simulink model "SAD_projectSamu"  (R2023b)
settings: Solver=ode4  StartTime=t0  StopTime=1000  FixedStep=t_step  RelTol=1e-3
model workspace (MAT data in the model file):
  N_order = 1
values from neighbouring files (symbols this model uses):
  A1 = importdata("igrfSg.txt")    [SAD_project_code.m]
  A2 = importdata("igrfSh.txt")    [SAD_project_code.m]
  A_1 = area_face(1)    [SAD_project_code.m]
  A_2 = area_face(2)    [SAD_project_code.m]
  A_3 = area_face(3)    [SAD_project_code.m]
  A_4 = area_face(4)    [SAD_project_code.m]
  A_5 = area_face(5)    [SAD_project_code.m]
  A_6 = area_face(6)    [SAD_project_code.m]
  alpha = [1/6 5/6]    [SAD_project_code.m]
  ARW = ARW*[1 1 1]'    [SAD_project_code.m]
  bias = bias*[1 1 1]'    [SAD_project_code.m]
  DCM_eci_per = rotationMatrix(rad2deg(i),rad2deg(OM), rad2deg(om))    [SAD_project_code.m]
  e = 0.0011241    [SAD_project_code.m]
  FS = 50000e-9    (= 5e-05)    [SAD_project_code.m]
  H0 = [g_10 g_11 h_11]'    [SAD_project_code.m]
  h_r_0 = [0,0,0]'    [SAD_project_code.m]
  horizon_cone_limit = deg2rad(350)    [SAD_project_code.m]
  I = 5/12.*diag([Ix Iy Iz])    [SAD_project_code.m]
  i = deg2rad(97.55)    [SAD_project_code.m]
  I_inv = inv(I)    [SAD_project_code.m]
  I_RW = 1e-2    (= 0.01)    [SAD_project_code.m]
  I_vector_RW = [I_RW I_RW I_RW]'    [SAD_project_code.m]
  inc_tot = sqrt(inc_lin^2 + inc_acc^2)    [SAD_project_code.m]
  InitialTrueAnomalyOfEarth = 0    [SAD_project_code.m]
  j_b = [0.001 0.005 0.001]'    [SAD_project_code.m]
  K1_point = lqr(A, B, Q, R)    [SAD_project_code.m]
  K1_slew = lqr(A,B, Q, R)    [SAD_project_code.m]
  K2_point = K1_point.^2/2    [SAD_project_code.m]
  K2_slew = K1_slew.^2/2    [SAD_project_code.m]
  K_detumbling = lqr(A,B,Q,R)    [SAD_project_code.m]
  matrix_RW_config = eye(3)    [SAD_project_code.m]
  matrix_RW_config_inv = inv(matrix_RW_config)    [SAD_project_code.m]
  mu_E = astroConstants(13)    [SAD_project_code.m]
  N_1 = BODY(1,:)    [SAD_project_code.m]
  N_2 = BODY(2,:)    [SAD_project_code.m]
  N_3 = BODY(3,:)    [SAD_project_code.m]
  N_4 = BODY(4,:)    [SAD_project_code.m]
  N_5 = BODY(5,:)    [SAD_project_code.m]
  N_6 = BODY(6,:)    [SAD_project_code.m]
  n_e = sqrt(mu_E/a^3)    [SAD_project_code.m]
  om = deg2rad(206.3209)    [SAD_project_code.m]
  OM = deg2rad(50.7464)    [SAD_project_code.m]
  p = a*(1-e^2)    [SAD_project_code.m]
  q0 = [0.1, -0.7, 0.51, 0.41]    [SAD_project_code.m]
  r_1 = r(1,:)    [SAD_project_code.m]
  r_2 = r(2,:)    [SAD_project_code.m]
  r_3 = r(3,:)    [SAD_project_code.m]
  r_4 = r(4,:)    [SAD_project_code.m]
  r_5 = r(5,:)    [SAD_project_code.m]
  r_6 = r(6,:)    [SAD_project_code.m]
  R_E = astroConstants(23)    [SAD_project_code.m]
  rho_d1 = 0.1    [SAD_project_code.m]
  rho_d2 = 0.1    [SAD_project_code.m]
  rho_d3 = 0.1    [SAD_project_code.m]
  rho_d4 = 0.1    [SAD_project_code.m]
  rho_d5 = 0.1    [SAD_project_code.m]
  rho_d6 = 0.1    [SAD_project_code.m]
  rho_s1 = rho_s(1)    [SAD_project_code.m]
  rho_s2 = rho_s(2)    [SAD_project_code.m]
  rho_s3 = rho_s(3)    [SAD_project_code.m]
  rho_s4 = rho_s(4)    [SAD_project_code.m]
  rho_s5 = rho_s(5)    [SAD_project_code.m]
  rho_s6 = rho_s(6)    [SAD_project_code.m]
  t_step = 0.01    [SAD_project_code.m]
  th0 = deg2rad(0)    [SAD_project_code.m]
  timeoflaunch = date2mjd2000(date0)    [SAD_project_code.m]
  torque_max = 0.8    [SAD_project_code.m]
  ts_sensor = 5*t_step    (= 0.05)    [SAD_project_code.m]
  w0 = [wx0 wy0 wz0]'    [SAD_project_code.m]
  w0_RW = [0 0 0]    [SAD_project_code.m]
  w_E = deg2rad(15.04)/60/60    [SAD_project_code.m]
  wMax_RW = 2*pi * RPM_max_RW / 60    (= 527.263967027)    [SAD_project_code.m]
libraries: matrix_library x43, dspindex x6, simulink x5, simulink_extras x4, sharedtransform x4, aerolibutil x2, vrlib x2, dspinverses x1
(part 1 of 4)
settings Model: PacingRate=0.100000  Creator=samue  LastModifiedBy=samue

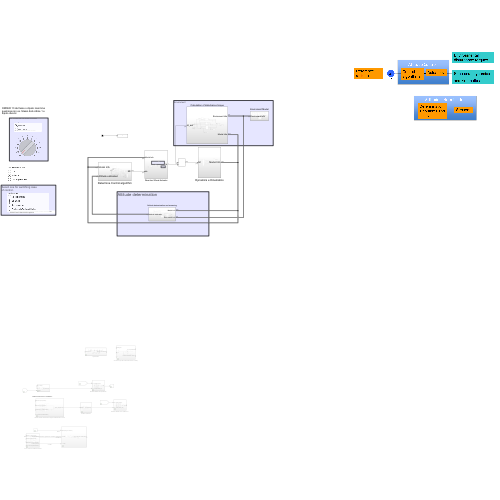
[thumbnail: Simulink's stored preview of the top-level diagram]
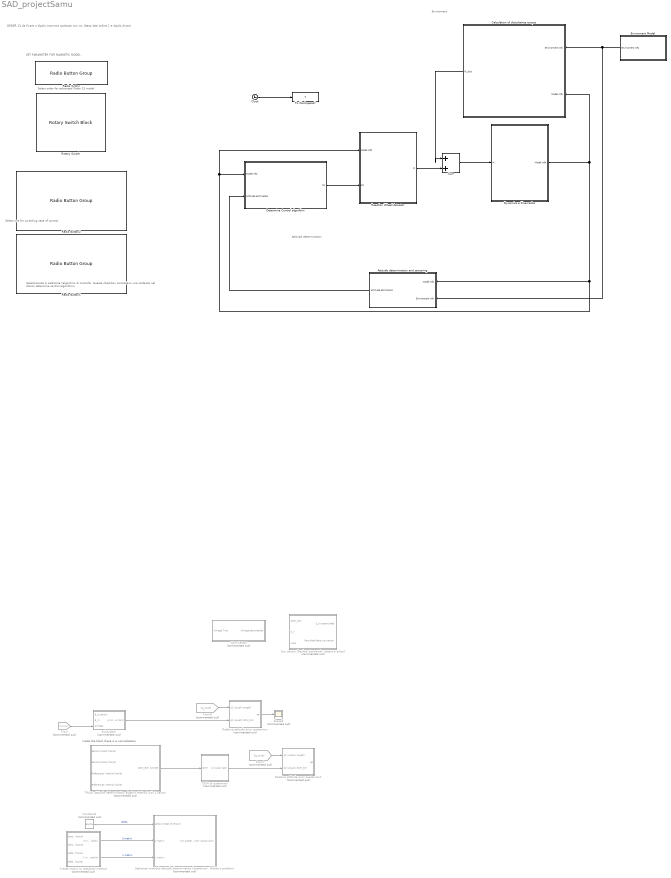
== system SAD_projectSamu ==
  note: ORDER 13 da fixare o dipolo insomma qualcosa non va. Stessi dati ordine 1 e dipolo diversi
  note: Select order for advanced Order 13 model
  note: SET PARAMETER FOR MAGNETIC MODEL
  note: Selezionando si seleziona l'algoritmo di controllo. Queste checkbox controllano una costante nel blocco determine control algorithmù
  note: Select one for switching case
      | of control.
  note: Attitude determination
  note: inside the block there is a normalisation
  note: Enviroment
  Attitude determination and sensoring : Subsystem
  Calculation of disturbance torque : Subsystem
  Clock : Clock
  Constant1 : Constant  Commented=on  Value=alpha
  Create matrix to statistical method : Subsystem  Commented=on
  DCM to quaternion : Subsystem  Commented=on
  Determine Control algorithm : Subsystem
  Dynamics e Kinematics : Subsystem
  Enviroment Model : Subsystem
  From : From  Commented=on  GotoTag=w_true
  From7 : From  Commented=on  GotoTag=q_true
  From8 : From  Commented=on  GotoTag=q_true
  Gyro Sensor : Subsystem  Commented=on
  Radio Button : RadioButtonGroup  LabelPosition=Hide  SelectedLabel=Dipole model  ButtonGroupName=Magnetic field
      settings: Values={{'Dipole model', 'Order 13 model'}, [0 1]}
  Radio Button1 : RadioButtonGroup  LabelPosition=Hide  SelectedLabel=De-tumble  ButtonGroupName=Control Mode
      settings: Values={{'No control mode', 'De-tumble', 'Slew maneuver', 'Pointing with 3 axis stabilization'}, [0 1 2 3]}
  Radio Button2 : RadioButtonGroup  LabelPosition=Hide  SelectedLabel=Statisitcal  ButtonGroupName=Attitude Determination
      settings: Values={{'Triad', 'Statisitcal', 'Only Magnetometer'}, [0 2 1]}
  Reaction Wheel Actuator : Subsystem
  Relative attitude error quaternion : Subsystem  Commented=on
  Relative attitude error quaternion1 : Subsystem  Commented=on
  Rotary Switch : RotarySwitchBlock  LabelPosition=Hide
      settings: Values={{'1', '2', '3', '4', '5', '6', '7', '8', '9', '10', '11', '12', '13'}, [1 2 3 4 5 6 7 8 9 10 11 12 13]}
  Scope3 : Scope  Commented=on
  "Statistical methods attitude determination (quaternion  Wabha’s problem) " : Subsystem  Commented=on
  Subsystem : Subsystem  Commented=on
  Sum : Sum  Inputs=|++
  Sun sensor (Da fare sistmando vettore e eclissi) : Subsystem  Commented=on
  TRIAD: Attitude determination algebric Method with 2 sensor : Subsystem  Commented=on
  To Workspace7 : ToWorkspace  VariableName=t  SampleTime=-1
  wires:
  Clock/1 -> To Workspace7/1
  Create matrix to statistical method/2(V matrix (inertia)) -> "Statistical methods attitude determination (quaternion  Wabha’s problem) "/3(v matrix)  "V matrix"
  Constant1/1 -> "Statistical methods attitude determination (quaternion  Wabha’s problem) "/1(alpha (weigh of sensor))  "alpha"
  Create matrix to statistical method/1(S matrix (body)) -> "Statistical methods attitude determination (quaternion  Wabha’s problem) "/2(s matrix)  "S matrix"
  TRIAD: Attitude determination algebric Method with 2 sensor/1(DCM_B/N  Att Det) -> DCM to quaternion/1(DCM)
  From/1 -> Subsystem/3(Omega)
  From8/1 -> Relative attitude error quaternion/1(q1 (usually target))
  Subsystem/1(q (scalar last)) -> Relative attitude error quaternion/2(q2 (usually DCM_bn))
  Relative attitude error quaternion/1(qe) -> Scope3/1
  DCM to quaternion/1(q (scalar last)) -> Relative attitude error quaternion1/2(q2 (usually DCM_bn))
  From7/1 -> Relative attitude error quaternion1/1(q1 (usually target))
  Reaction Wheel Actuator/1(M) -> Sum/2
  Sum/1 -> Dynamics e Kinematics/1(M)
  Enviroment Model/1(Enviroment Info) -> Attitude determination and sensoring/2(Enviroment info), Calculation of disturbance torque/1(Enviroment Info)
  Calculation of disturbance torque/1(M_dist) -> Sum/1
  Determine Control algorithm/1(Mc) -> Reaction Wheel Actuator/2(Mc)
  Dynamics e Kinematics/1(Model Info) -> Calculation of disturbance torque/2(Model Info), Determine Control algorithm/1(Model Info), Reaction Wheel Actuator/1(Model Info), Attitude determination and sensoring/1(Model Info)
  Attitude determination and sensoring/1(Attitude estimation) -> Determine Control algorithm/2(Attitude estimated)

== system SAD_projectSamu/Attitude determination and sensoring ==
  Model Info : Inport
  Enviroment info : Inport  Port=2
  Bus Selector : BusSelector  OutputSignals=B_N,r_n
  Bus Selector1 : BusSelector  OutputSignals=w_b true,DCM_BN,q_b True
  Demux : Demux
  Demux1 : Demux  Outputs=3
  Display : Display
  Horizon Sensor : Subsystem
  MAG-3  Magnetometer1 : Subsystem
  Relative attitude error quaternion2 : Subsystem
  Reshape3 : Reshape
  "SCOPE ERROR ATTITUTE ESTIMATION RESPECT TO DCM_BN TRUE " : Scope  NumInputPorts=4
  "SCOPE ERROR w estimated RESPECT TO w TRUE " : Scope  NumInputPorts=3
  Subsystem1 : Subsystem
  Subtract : Sum  Inputs=+-
  To Workspace5 : ToWorkspace  VariableName=b_sensor  SampleTime=-1
  Transpose : Math  Operator=transpose
  Out Bus Element2 : Outport  PortName=Attitude estimation  Element=q estimated
  Out Bus Element1 : Outport  PortName=Attitude estimation  Element=w estimated
  wires:
  MAG-3  Magnetometer1/2(B_n) -> Subsystem1/3(B_N)
  Horizon Sensor/3(Falg IsEarthVisible) -> Subsystem1/6(Flag IsEarthVisible)
  Horizon Sensor/1(Perturbed data Horizon) -> Subsystem1/4(Horizon_b sensor)  "R_b perturbed sensor"
  Horizon Sensor/2(R_N Horizon) -> Subsystem1/5(Horizon_N)
  MAG-3  Magnetometer1/1(B_b perturbed sensor) -> Subsystem1/2(B_b sensor), Reshape3/1
  Bus Selector/1 -> Transpose/1  "<B_N>"
  Enviroment info/1 -> Bus Selector/1
  Bus Selector/2 -> Horizon Sensor/2(R_N)  "<r_n>"
  Bus Selector1/2 -> Horizon Sensor/1(DCM_B/N), MAG-3  Magnetometer1/1(DCM_B/N)  "<DCM_BN>"
  Reshape3/1 -> To Workspace5/1
  Model Info/1 -> Bus Selector1/1
  Transpose/1 -> MAG-3  Magnetometer1/2(B_N)
  Demux/1 -> "SCOPE ERROR ATTITUTE ESTIMATION RESPECT TO DCM_BN TRUE "/1
  Demux/3 -> "SCOPE ERROR ATTITUTE ESTIMATION RESPECT TO DCM_BN TRUE "/3
  Relative attitude error quaternion2/1(qe) -> Demux/1
  Demux/4 -> "SCOPE ERROR ATTITUTE ESTIMATION RESPECT TO DCM_BN TRUE "/4
  Bus Selector1/1 -> Subtract/1, Subsystem1/1(w_true)  "<w_b true>"
  Demux/2 -> "SCOPE ERROR ATTITUTE ESTIMATION RESPECT TO DCM_BN TRUE "/2
  Bus Selector1/3 -> Relative attitude error quaternion2/1(q1 (usually Target))  "<q_b True>"
  Subtract/1 -> Demux1/1
  Demux1/2 -> "SCOPE ERROR w estimated RESPECT TO w TRUE "/2
  Demux1/1 -> "SCOPE ERROR w estimated RESPECT TO w TRUE "/1
  Demux1/3 -> "SCOPE ERROR w estimated RESPECT TO w TRUE "/3
  Subsystem1/1(q estimated) -> Out Bus Element2/1, Display/1, Relative attitude error quaternion2/2(q2 (Estimated))
  Subsystem1/2(w estimated) -> Out Bus Element1/1, Subtract/2

== system SAD_projectSamu/Calculation of disturbance torque ==
  Enviroment Info : Inport
  Model Info : Inport  Port=2
  Bus Selector : BusSelector  OutputSignals=r_n,S_N,B_N
  Bus Selector1 : BusSelector  OutputSignals=DCM_BL,DCM_BN
  Constant : Constant  Value=I
  Extract Diagonal : matrix_library/Extract Diagonal
      settings: LibrarySourceBlock=|
      | simulink/Matrix
      | Operations/Extract Diagonal
  M of gravity gradient1 : Subsystem
  Magnetic Torque : Subsystem
  Matrix Multiply : Product  Multiplication=Matrix(*)
  Reshape{,1..2,4} (4 alike) : Reshape
  Solar pressure on 6 faces : Subsystem
  Sum : Sum  Inputs=|+++
  Terminator : Terminator
  To Workspace1 : ToWorkspace  VariableName=M_b  SampleTime=-1
  To Workspace2 : ToWorkspace  VariableName=M_dist  SampleTime=-1
  To Workspace3 : ToWorkspace  VariableName=M_GG  SampleTime=-1
  To Workspace6 : ToWorkspace  VariableName=bn  SampleTime=-1
  To Workspace8 : ToWorkspace  VariableName=M_SRP  SampleTime=-1
  j_b : Constant  Value=j_b
  M_dist : Outport
  wires:
  j_b/1 -> Magnetic Torque/1(j_b)
  Magnetic Torque/1(M_b) -> Sum/3, Reshape1/1
  Sum/1 -> Reshape2/1, M_dist/1
  Reshape/1 -> To Workspace8/1
  Reshape1/1 -> To Workspace1/1
  M of gravity gradient1/1(GravityGradient_M) -> To Workspace3/1, Sum/1
  Solar pressure on 6 faces/2(Ftot_SP) -> Terminator/1
  Solar pressure on 6 faces/1(Mtot_SP) -> Reshape/1
  Extract Diagonal/1 -> M of gravity gradient1/1(Inertia Vector)
  Reshape4/1 -> To Workspace6/1
  Matrix Multiply/1 -> Reshape4/1, Magnetic Torque/2(B_b)  "B_b"
  Enviroment Info/1 -> Bus Selector/1
  Constant/1 -> Extract Diagonal/1
  Bus Selector/1 -> M of gravity gradient1/3(r_N), Solar pressure on 6 faces/2("r_N ")  "<r_n>"
  Bus Selector/2 -> Solar pressure on 6 faces/3(S_N)  "<S_N>"
  Bus Selector/3 -> Matrix Multiply/1  "<B_N>"
  Model Info/1 -> Bus Selector1/1
  Bus Selector1/2 -> Matrix Multiply/2, Solar pressure on 6 faces/1(DCM_BN)  "<DCM_BN>"
  Bus Selector1/1 -> M of gravity gradient1/2(A_B/L)  "<DCM_BL>"
  Reshape2/1 -> To Workspace2/1

== system SAD_projectSamu/Create matrix to statistical method ==
  Sensor1 (body frame) : Inport
  Sensor2 (body frame) : Inport  Port=2
  Reference1 (Inertial frame) : Inport  Port=3
  Reference2 (Inertial frame) : Inport  Port=4
  Matrix Concatenate1 : Concatenate  Mode=Multidimensional array  ConcatenateDimension=2
  Matrix Concatenate2 : Concatenate  Mode=Multidimensional array  ConcatenateDimension=2
  Normalize Vector1 : Subsystem
  Normalize Vector2 : Subsystem
  Normalize Vector3 : Subsystem
  Normalize Vector4 : Subsystem
  S matrix (body) : Outport
  V matrix (inertia) : Outport  Port=2
  wires:
  Matrix Concatenate1/1 -> V matrix (inertia)/1
  Normalize Vector1/1(Versor) -> Matrix Concatenate2/1
  Normalize Vector2/1(Versor) -> Matrix Concatenate2/2
  Normalize Vector4/1(Versor) -> Matrix Concatenate1/2
  Normalize Vector3/1(Versor) -> Matrix Concatenate1/1
  Matrix Concatenate2/1 -> S matrix (body)/1
  Reference1 (Inertial frame)/1 -> Normalize Vector3/1(Vector)
  Reference2 (Inertial frame)/1 -> Normalize Vector4/1(Vector)
  Sensor1 (body frame)/1 -> Normalize Vector1/1(Vector)
  Sensor2 (body frame)/1 -> Normalize Vector2/1(Vector)

== system SAD_projectSamu/DCM to quaternion ==
  DCM : Inport
  Constant : Constant
  Divide : Product  Inputs=*/
  Extract Diagonal : matrix_library/Extract Diagonal
      settings: LibrarySourceBlock=|
      | simulink/Matrix
      | Operations/Extract Diagonal
  Gain : Gain  Gain=0.5
  Gain1 : Gain  Gain=[0 0 0; 0 0 1; 0 -1 0]
  Gain2 : Gain  Gain=[0 0 -1; 0 0 0; 1 0 0]
  Gain3 : Gain  Gain=[0 1 0; -1 0 0; 0 0 0]
  Gain4 : Gain  Gain=4
  Normalize Vector1 : Subsystem
  Sqrt : Sqrt
  Sum : Sum  Inputs=|++
  Sum of Elements{,1..3} (4 alike) : Sum  Inputs=+
  Vector Concatenate : Concatenate  NumInputs=3
  Vector Concatenate1 : Concatenate
  q (scalar last) : Outport
  wires:
  Extract Diagonal/1 -> Sum of Elements/1
  Sum of Elements/1 -> Sum/1
  Constant/1 -> Sum/2
  Sum/1 -> Sqrt/1
  Sqrt/1 -> Gain/1
  DCM/1 -> Gain1/1, Gain2/1, Gain3/1, Extract Diagonal/1
  Gain2/1 -> Sum of Elements1/1
  Sum of Elements1/1 -> Vector Concatenate/2
  Gain1/1 -> Sum of Elements2/1
  Sum of Elements2/1 -> Vector Concatenate/1
  Sum of Elements3/1 -> Vector Concatenate/3
  Gain3/1 -> Sum of Elements3/1
  Vector Concatenate/1 -> Divide/1
  Gain/1 -> Vector Concatenate1/2, Gain4/1
  Gain4/1 -> Divide/2
  Divide/1 -> Vector Concatenate1/1
  Vector Concatenate1/1 -> Normalize Vector1/1(Vector)
  Normalize Vector1/1(Versor) -> q (scalar last)/1

== system SAD_projectSamu/Determine Control algorithm ==
  Model Info : Inport
  Attitude estimated : Inport  Port=2
  Bus Selector : BusSelector  OutputSignals=q estimated
  Constant2 : Constant
  Demux : Demux
  Demux4 : Demux
  Demux5 : Demux
  Merge : Merge  Inputs=4
  Merge1 : Merge
  Mux{4..7} (4 alike) : Mux  Inputs=2
  Relative attitude error quaternion3 : Subsystem
  Saturation : Saturate  LowerLimit=-torque_max
  Scope : Scope  NumInputPorts=4
  Scope1 : Scope  NumInputPorts=4
  Switch Case : SwitchCase  CaseConditions={1,2,3}
  Switch Case Action 3 axis stabilization Algorithm : Subsystem  TreatAsAtomicUnit=on
  Switch Case Action Detumle Algorithm : Subsystem  TreatAsAtomicUnit=on
  Switch Case Action Mc = 0 : Subsystem  TreatAsAtomicUnit=on
  Switch Case Action Slew Maneuver Algorithm : Subsystem  TreatAsAtomicUnit=on
  Zero-Order Hold : ZeroOrderHold  SampleTime=5*ts_sensor
  Zero-Order Hold1 : ZeroOrderHold  SampleTime=5*ts_sensor
  Mc : Outport
  wires:
  Switch Case/2 -> Switch Case Action Slew Maneuver Algorithm/Action  "slew maneuver"
  Switch Case/1 -> Switch Case Action Detumle Algorithm/Action  "Detumble case"
  Switch Case Action Slew Maneuver Algorithm/1(Mc) -> Merge/2
  Switch Case/3 -> Switch Case Action 3 axis stabilization Algorithm/Action  "pointing with 3 axis stabilization"
  Switch Case Action Mc = 0/1(Output) -> Merge/4
  Constant2/1 -> Switch Case/1
  Switch Case Action Detumle Algorithm/1(Out1) -> Merge/1
  Switch Case Action 3 axis stabilization Algorithm/1(Mc) -> Merge/3
  Switch Case/4 -> Switch Case Action Mc = 0/Action  "Default: Contol moment == 0"
  Merge/1 -> Saturation/1  "Control Moment"
  Model Info/1 -> Zero-Order Hold1/1
  Attitude estimated/1 -> Zero-Order Hold/1
  Demux4/1 -> Mux4/2
  Demux4/4 -> Mux7/2
  Demux5/3 -> Mux6/1
  Demux5/4 -> Mux7/1
  Mux5/1 -> Scope1/2
  Merge1/1 -> Demux5/1, Relative attitude error quaternion3/1(q1 (usually Target))  "q target"
  Mux6/1 -> Scope1/3
  Mux7/1 -> Scope1/4
  Demux4/3 -> Mux6/2
  Demux5/2 -> Mux5/1
  Demux4/2 -> Mux5/2
  Mux4/1 -> Scope1/1
  Demux5/1 -> Mux4/1
  Switch Case Action 3 axis stabilization Algorithm/2(q target) -> Merge1/1
  Bus Selector/1 -> Relative attitude error quaternion3/2(q2 (Estimated)), Demux4/1  "<q estimated>"
  Switch Case Action Slew Maneuver Algorithm/2(q target) -> Merge1/2
  Relative attitude error quaternion3/1(qe) -> Demux/1
  Demux/1 -> Scope/1
  Demux/2 -> Scope/2
  Demux/3 -> Scope/3
  Demux/4 -> Scope/4
  Zero-Order Hold1/1 -> Switch Case Action Slew Maneuver Algorithm/1(Model info), Switch Case Action 3 axis stabilization Algorithm/1(Model info)
  Zero-Order Hold/1 -> Switch Case Action 3 axis stabilization Algorithm/2(InBus), Switch Case Action Detumle Algorithm/1(Attitude estimated), Switch Case Action Slew Maneuver Algorithm/2(Attitude estimated), Bus Selector/1
  Saturation/1 -> Mc/1

== system SAD_projectSamu/Dynamics e Kinematics ==
  M : Inport
  Attitude error GG : Subsystem
  Constant : Constant  Value=I_inv
  Constant6 : Constant  Value=q0
  DCM composition from quaternions 1 : Subsystem  AncestorBlock=LibrarySAD5/DCM composition from quaternions
  Inertia Matrix : Constant  Value=I  VectorParams1D=off
  Initial Condition W : Constant  Value=w0
  Kinematics quaternion2 : Subsystem
  Reshape : Reshape
  Reshape1 : Reshape
  Single spin dynamics : Subsystem  AncestorBlock=My_library/Single spin dynamics
  Terminator1 : Terminator
  To Workspace2 : ToWorkspace  VariableName=wb  SampleTime=-1
  To Workspace4 : ToWorkspace  VariableName=w  SampleTime=-1
  Transpose : Math  Operator=transpose
  Out Bus Element : Outport  PortName=Model Info  Element=w_b true
  Out Bus Element1 : Outport  PortName=Model Info  Element=Ang vel error
  Out Bus Element2 : Outport  PortName=Model Info  Element=DCM_BL
  Out Bus Element3 : Outport  PortName=Model Info  Element=q_b True
  Out Bus Element4 : Outport  PortName=Model Info  Element=DCM_BN
  Out Bus Element5 : Outport  PortName=Model Info  Element=A_L/N
  wires:
  Single spin dynamics/1(Omega) -> Transpose/1, Attitude error GG/1(w), Reshape1/1, Kinematics quaternion2/1(omega)  "w_b true"
  M/1 -> Single spin dynamics/4(M)
  Constant/1 -> Single spin dynamics/1(Inertia matrix inverse)
  Inertia Matrix/1 -> Single spin dynamics/2(Inertia matrix)
  Initial Condition W/1 -> Single spin dynamics/3(Omega_0)
  Constant6/1 -> Kinematics quaternion2/2(q0)
  Kinematics quaternion2/1(q) -> DCM composition from quaternions 1/1(q(4x1)), Out Bus Element3/1  "q_b True"
  Reshape1/1 -> To Workspace4/1
  Kinematics quaternion2/2(q^(-1)) -> Terminator1/1
  DCM composition from quaternions 1/1(DCM) -> Out Bus Element4/1, Attitude error GG/2(DCM_B/N)  "DCM_BN"
  Attitude error GG/1(Ang Vel Error) -> Out Bus Element1/1, Reshape/1  "Ang vel error"
  Attitude error GG/2(DCM_B/L) -> Out Bus Element2/1
  Reshape/1 -> To Workspace2/1
  Transpose/1 -> Out Bus Element/1
  Attitude error GG/3(A_L/N) -> Out Bus Element5/1

== system SAD_projectSamu/Enviroment Model ==
  Bus Creator : BusCreator  Inputs=3
  Constant4 : Constant  Value=th0
  Magnetic Field : Subsystem
  Sun Position in Earth Centred Equatorial Inertial RF : Subsystem
  To Workspace : ToWorkspace  VariableName=r_n  SampleTime=-1
  two-body Keplerian dynamics ECI : Subsystem
  Enviroment Info : Outport
  wires:
  Constant4/1 -> two-body Keplerian dynamics ECI/1(th0)
  Sun Position in Earth Centred Equatorial Inertial RF/1(s_N) -> Bus Creator/2  "S_N"
  two-body Keplerian dynamics ECI/1(r_n) -> Magnetic Field/1(r_N), Bus Creator/1, To Workspace/1  "r_n"
  Magnetic Field/1(B_N) -> Bus Creator/3  "B_N"
  Bus Creator/1 -> Enviroment Info/1

== system SAD_projectSamu/Gyro Sensor ==
  Omega True : Inport
  Band-Limited White Noise : simulink/Sources/Band-Limited White Noise  Cov=[0.00001]  Ts=0.1  seed=[23341]
  Constant : Constant  Value=ARW  VectorParams1D=off
  Constant1 : Constant  Value=bias  VectorParams1D=off
  Sum : Sum  Inputs=|++
  Sum1 : Sum  Inputs=|++
  Sum2 : Sum  Inputs=|++
  Zero-Order Hold : ZeroOrderHold  SampleTime=-1
  Omega perturbated : Outport
  wires:
  Zero-Order Hold/1 -> Sum/1
  Sum2/1 -> Omega perturbated/1
  Sum1/1 -> Sum2/1
  Sum/1 -> Sum1/1
  Omega True/1 -> Zero-Order Hold/1
  Constant1/1 -> Sum2/2
  Band-Limited White Noise/1 -> Sum/2
  Constant/1 -> Sum1/2

== system SAD_projectSamu/Reaction Wheel Actuator ==
  note: W integration
  note: MAIN INTEGRATION
  BusElementIn : Inport  PortName=Model Info  Element=w_b true
  Mc : Inport  Port=2
  Calculatate wRW in base of saturation : Subsystem
  Constant3 : Constant  Value=I_vector_RW
  Constant5 : Constant  Value=h_r_0  VectorParams1D=off
  Constant6 : Constant  Value=matrix_RW_config  VectorParams1D=off
  Constant8 : Constant  Value=matrix_RW_config_inv  VectorParams1D=off
  Constant9 : Constant  Value=w0_RW
  Cross Product : matrix_library/Cross Product
  Divide : Product  Inputs=*/
  Gain : Gain  Gain=-1
  Integrator : Integrator  InitialConditionSource=external
  Integrator1 : Integrator  InitialConditionSource=external
  Matrix Multiply : Product  Multiplication=Matrix(*)
  Matrix Multiply1 : Product  Multiplication=Matrix(*)
  Reshape : Reshape
  Reshape4 : Reshape
  Saturation : Saturate  UpperLimit=wMax_RW*I_RW  LowerLimit=-wMax_RW*I_RW
  Subsystem1 : Subsystem
  Sum : Sum  Inputs=|++
  To Workspace1 : ToWorkspace  VariableName=wr  SampleTime=-1
  To Workspace6 : ToWorkspace  VariableName=M_actuator  SampleTime=-1
  detect if the RW is saturated (output == 1 isSaturated) : Subsystem
  M : Outport
  wires:
  Matrix Multiply1/1 -> Integrator/1, Divide/1  "h_r dot"
  Constant6/1 -> Matrix Multiply/1
  Cross Product/1 -> Sum/2
  Constant8/1 -> Gain/1
  Sum/1 -> Matrix Multiply1/2
  detect if the RW is saturated (output == 1 isSaturated)/2(flag RW2) -> Subsystem1/2(flag RW2 (1 is saturated)), Calculatate wRW in base of saturation/3(flag RW2 (1 is saturated))  "flag RW2 (1 is saturated)"
  Calculatate wRW in base of saturation/1(wRW) -> Reshape/1
  Matrix Multiply/1 -> Cross Product/2
  Constant5/1 -> Integrator/2
  Constant3/1 -> Divide/2
  Gain/1 -> Matrix Multiply1/1
  Mc/1 -> Subsystem1/4(Mc), Sum/1
  Saturation/1 -> Matrix Multiply/2
  Integrator1/1 -> Calculatate wRW in base of saturation/1(wRW integrated), detect if the RW is saturated (output == 1 isSaturated)/1(w)  "wRW integrated"
  Constant9/1 -> Integrator1/2
  Divide/1 -> Integrator1/1  "wRW dot"
  Integrator/1 -> Saturation/1  "h_r"
  detect if the RW is saturated (output == 1 isSaturated)/3(flag RW3) -> Subsystem1/3(flag RW3 (1 is saturated)), Calculatate wRW in base of saturation/4(flag RW3 (1 is saturated))  "flag RW3 (1 is saturated)"
  detect if the RW is saturated (output == 1 isSaturated)/1(flag RW1) -> Subsystem1/1(flag RW1 (1 is saturated)), Calculatate wRW in base of saturation/2(flag RW1 (1 is saturated))  "flag RW1 (1 is saturated)"
  Reshape/1 -> To Workspace1/1
  Subsystem1/1(M) -> Reshape4/1, M/1
  Reshape4/1 -> To Workspace6/1
  BusElementIn/1 -> Cross Product/1

== system SAD_projectSamu/Relative attitude error quaternion ==
  q1 (usually target) : Inport
  q2 (usually DCM_bn) : Inport  Port=2
  Demux : Demux
  Gain1 : Gain  Gain=[0,0,0,-1; 0,0,1,0; 0,-1,0 0; 1,0,0,0]
  Gain2 : Gain  Gain=[0, 0, -1 ,0; 0, 0 ,0 ,-1; 1, 0, 0, 0; 0 1, 0, 0]
  Gain3 : Gain  Gain=[0 1 0 0; -1 0 0 0; 0 0 0 -1; 0 0 1 0]
  Gain4 : Gain  Gain=eye(4)
  Matrix Multiply : Product  Multiplication=Matrix(*)
  Sum1 : Sum  Inputs=++++
  qe : Outport
  wires:
  Gain1/1 -> Sum1/1
  Demux/2 -> Gain2/1
  Gain3/1 -> Sum1/3
  Demux/1 -> Gain1/1
  Sum1/1 -> Matrix Multiply/1
  Demux/3 -> Gain3/1
  Gain4/1 -> Sum1/4
  Gain2/1 -> Sum1/2
  Demux/4 -> Gain4/1
  q2 (usually DCM_bn)/1 -> Matrix Multiply/2
  Matrix Multiply/1 -> qe/1
  q1 (usually target)/1 -> Demux/1

== system SAD_projectSamu/Relative attitude error quaternion1 ==
  q1 (usually target) : Inport
  q2 (usually DCM_bn) : Inport  Port=2
  Demux : Demux
  Gain1 : Gain  Gain=[0,0,0,-1; 0,0,1,0; 0,-1,0 0; 1,0,0,0]
  Gain2 : Gain  Gain=[0, 0, -1 ,0; 0, 0 ,0 ,-1; 1, 0, 0, 0; 0 1, 0, 0]
  Gain3 : Gain  Gain=[0 1 0 0; -1 0 0 0; 0 0 0 -1; 0 0 1 0]
  Gain4 : Gain  Gain=eye(4)
  Matrix Multiply : Product  Multiplication=Matrix(*)
  Sum1 : Sum  Inputs=++++
  qe : Outport
  wires:
  Gain1/1 -> Sum1/1
  Demux/2 -> Gain2/1
  Gain3/1 -> Sum1/3
  Demux/1 -> Gain1/1
  Sum1/1 -> Matrix Multiply/1
  Demux/3 -> Gain3/1
  Gain4/1 -> Sum1/4
  Gain2/1 -> Sum1/2
  Demux/4 -> Gain4/1
  q2 (usually DCM_bn)/1 -> Matrix Multiply/2
  Matrix Multiply/1 -> qe/1
  q1 (usually target)/1 -> Demux/1

== system SAD_projectSamu/Statistical methods attitude determination (quaternion  Wabha’s problem)  ==
  note: In questo blocco ci sono altri metodi per il calcolo di q
  note: BLOCCO DA SISTEMARE SCEGLIENDO UNA SOLUZIONE
  note: Resolve linear system:
      | (𝑆 − σI)𝑞 + zq_4 = 𝜆_(MAX)*𝑞
      | 𝑧'𝑞 + σ*q_4 = 𝜆_(MAX)*𝑞_4
      |
      | Calculate eigenvalue (in the theory we assumed that lambda_max = 1)
  note: 𝐾 = [ (𝑆 − σI), 𝑧
      | 𝑧 ' 𝜎 ]
  note: 𝑧 = [𝑏23 − 𝑏32 , b31 − 𝑏13 , b12 − 𝑏21] '
  alpha (weigh of sensor) : Inport
  s matrix : Inport  Port=2
  v matrix : Inport  Port=3
  Adjoint of 3x3 Matrix : aerolibutil/Adjoint of 3x3 Matrix
  Blocco da convertire in formato simulink. Ho trovato 3 soluzioni differenti al proble : MATLAB Function  TreatAsAtomicUnit=on
  For Iterator Subsystem to calculate B matrix : Subsystem  TreatAsAtomicUnit=on
  Gain : Gain  Gain=eye(3)
  Matrix Concatenate : Concatenate  Mode=Multidimensional array  ConcatenateDimension=2
  Matrix Concatenate1 : Concatenate  Mode=Multidimensional array
  Matrix trace : Subsystem
  Subtract : Sum  Inputs=+-
  Sum : Sum  Inputs=|++
  Transpose : Math  Operator=transpose
  Transpose2 : Math  Operator=transpose
  Vector Concatenate1 : Concatenate
  Vector z : Subsystem
  q in quaternion (scalar last) : Outport
  wires:
  Transpose/1 -> Sum/2
  For Iterator Subsystem to calculate B matrix/1(B matrix) -> Vector z/1(B), Matrix trace/1(Matrix), Transpose/1, Sum/1  "B matrix"
  Sum/1 -> Adjoint of 3x3 Matrix/1, Blocco da convertire in formato simulink. Ho trovato 3 soluzioni differenti al proble/2(S), Subtract/1  "matrix S"
  Gain/1 -> Subtract/2
  Matrix trace/1(trace) -> Vector Concatenate1/2, Gain/1  "sigma = tr(B)"
  Matrix Concatenate/1 -> Matrix Concatenate1/1
  Vector Concatenate1/1 -> Transpose2/1
  Vector z/1(z) -> Vector Concatenate1/1, Matrix Concatenate/2
  Transpose2/1 -> Matrix Concatenate1/2
  Subtract/1 -> Matrix Concatenate/1  "S - sigma*eye(3)"
  alpha (weigh of sensor)/1 -> For Iterator Subsystem to calculate B matrix/1(alpha)
  v matrix/1 -> For Iterator Subsystem to calculate B matrix/3(v matrix)
  s matrix/1 -> For Iterator Subsystem to calculate B matrix/2(s matrix)
  Blocco da convertire in formato simulink. Ho trovato 3 soluzioni differenti al proble/1(q) -> q in quaternion (scalar last)/1  "q in quaternion (scalar last)"
  Adjoint of 3x3 Matrix/1 -> Blocco da convertire in formato simulink. Ho trovato 3 soluzioni differenti al proble/3(Sadj)
  Matrix Concatenate1/1 -> Blocco da convertire in formato simulink. Ho trovato 3 soluzioni differenti al proble/1(K)  "K matrix"

== system SAD_projectSamu/Subsystem ==
  B_b sensor : Inport
  B_N : Inport  Port=2
  Omega : Inport  Port=3
  Cross Product4 : matrix_library/Cross Product
  DCM to quaternion : Subsystem
  Divide : Product  Inputs=*/
  Gain3 : Gain  Gain=1/ts_sensor
  Matrix Multiply2 : Product  Multiplication=Matrix(*)
  Norm vector : Subsystem  AncestorBlock=LibrarySAD5/Normalize Vector1
  Normalize Vector1 : Subsystem
  Normalize Vector5 : Subsystem
  Scope : Scope
  Square : Math  Operator=square
  Subsystem : Subsystem
  Subsystem1 : Subsystem
  Subtract3 : Sum  Inputs=+-
  Transpose : Math  Operator=transpose
  Unit Delay2 : UnitDelay  InitialCondition=[1,0,0]'  SampleTime=-1  HasFrameUpgradeWarning=on
  Zero-Order Hold : ZeroOrderHold  SampleTime=ts_sensor
  time derivative : Subsystem
  q (scalar last) : Outport
  wires:
  time derivative/1(B_b dot Versor) -> Norm vector/1(Vector), Unit Delay2/1, Cross Product4/1  "B_b dot"
  Unit Delay2/1 -> Cross Product4/2
  Norm vector/1(Norm) -> Square/1
  Cross Product4/1 -> Divide/1
  Square/1 -> Divide/2
  Divide/1 -> Gain3/1
  Matrix Multiply2/1 -> DCM to quaternion/1(DCM)
  DCM to quaternion/1(q (scalar last)) -> q (scalar last)/1
  Normalize Vector1/1(Versor) -> Subsystem/1(B_b versor)  "B_b versor"
  Subsystem/1(b_matrix) -> Matrix Multiply2/1
  B_N/1 -> Zero-Order Hold/1
  Normalize Vector5/1(Versor) -> Subsystem1/1(B_N versor)
  Subsystem1/1(r_matrix) -> Matrix Multiply2/2
  Zero-Order Hold/1 -> Normalize Vector5/1(Vector)
  Omega/1 -> Transpose/1
  Subtract3/1 -> Scope/1
  Gain3/1 -> Subtract3/2
  Transpose/1 -> Subtract3/1
  B_b sensor/1 -> time derivative/1(B_b), Normalize Vector1/1(Vector)

== system SAD_projectSamu/Sun sensor (Da fare sistmando vettore e eclissi) ==
  note: SUN SENSOR DA RIFINIRE, ma Utilizzabile
      | -> Modellare non rilevamento sole (esempio eclissi)
      | -> Modellare albedo terra/luna per riflessi
      | -> Sistemare distrubi basandosi su sensore reale
  DCM_B/N : Inport
  S_n : Inport  Port=2
  Input : Inport  Port=3
  Band-Limited White Noise : simulink/Sources/Band-Limited White Noise  Cov=5e9*[1 1 1]  Ts=ts_sensor  seed=[23341]
  Normalize Vector1 : Subsystem
  Rotation in body frame : Product  Multiplication=Matrix(*)
  Rotation in body frame1 : Product  Multiplication=Matrix(*)
  Sum : Sum  Inputs=|++
  Zero-Order Hold : ZeroOrderHold  SampleTime=ts_sensor
  S_b unperturbed : Outport
  Perturbed data sun sensor : Outport  Port=2
  wires:
  Band-Limited White Noise/1 -> Sum/2
  DCM_B/N/1 -> Rotation in body frame/1, Rotation in body frame1/1
  S_n/1 -> Zero-Order Hold/1, Normalize Vector1/1(Vector)
  Normalize Vector1/1(Versor) -> Rotation in body frame/2
  Zero-Order Hold/1 -> Rotation in body frame1/2
  Rotation in body frame1/1 -> Sum/1
  Rotation in body frame/1 -> S_b unperturbed/1
  Sum/1 -> Perturbed data sun sensor/1

== system SAD_projectSamu/TRIAD: Attitude determination algebric Method with 2 sensor ==
  note: 𝑉^(-1) = 𝑉';
      | 𝐴 = 𝑆𝑉^(-1) = 𝑆𝑉'
  note: 𝑣1 = 𝑎;
      | 𝑣2 = (𝑎 ∧ 𝑏)/|𝑎 ∧ 𝑏|;
      | 𝑣3 = 𝑎 ∧ 𝑣2
  note: S1 = 𝑝;
      | 𝑠2 = (𝑝 ∧ 𝑞)/(|𝑝 ∧ 𝑞|);
      | 𝑠3 = 𝑝 ∧ 𝑠2
  Sensor1 (body frame) : Inport
  Sensor2 (body frame) : Inport  Port=2
  Reference1 (Inertial frame) : Inport  Port=3
  Reference2 (Inertial frame) : Inport  Port=4
  Matrix Multiply : Product  Multiplication=Matrix(*)
  Normalize Vector1 : Subsystem
  Normalize Vector2 : Subsystem
  Normalize Vector3 : Subsystem
  Normalize Vector4 : Subsystem
  Subsystem : Subsystem
  Subsystem1 : Subsystem
  Transpose : Math  Operator=transpose
  DCM_B/N  Att Det : Outport
  wires:
  Sensor1 (body frame)/1 -> Normalize Vector2/1(Vector)  "q"
  Sensor2 (body frame)/1 -> Normalize Vector3/1(Vector)  "p"
  Subsystem/1("Matrix S Measurements ") -> Matrix Multiply/1  "Matrix S Measurements (body frame)"
  Normalize Vector2/1(Versor) -> Subsystem/1(versor p (body frame))
  Normalize Vector3/1(Versor) -> Subsystem/2(versor q (body frame))
  Reference2 (Inertial frame)/1 -> Normalize Vector4/1(Vector)  "b"
  Reference1 (Inertial frame)/1 -> Normalize Vector1/1(Vector)  "a"
  Subsystem1/1("Matrix V certain model ") -> Transpose/1  "Matrix V (inertial frame)"
  Normalize Vector4/1(Versor) -> Subsystem1/2(versor b (inertial))
  Matrix Multiply/1 -> DCM_B/N  Att Det/1  "DCM_B/N from attirude determination"
  Transpose/1 -> Matrix Multiply/2
  Normalize Vector1/1(Versor) -> Subsystem1/1(versor a (inertial))

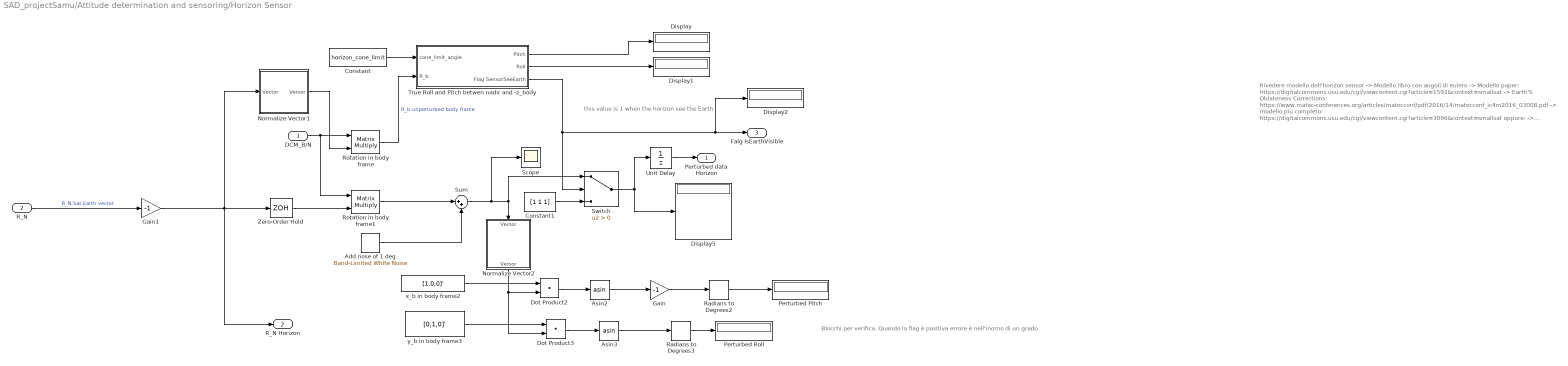
== system SAD_projectSamu/Attitude determination and sensoring/Horizon Sensor ==
  note: this value is 1 when the horizon see the Earth
  note: Rivedere modello dell'horizon sensor
      | -> Modello libro con angoli di eulero
      | -> Modello paper: https://digitalcommons.usu.edu/cgi/viewcontent.cgi?article=1592&context=smallsat
      | -> Earth’S Oblateness Corrections: https://www.matec-conferences.org/articles/matecconf/pdf/2016/14/matecconf_ic4m2016_03008.pdf
      | -> modello più completo: https://digitalcommons.usu.edu/cgi/viewcontent.cgi?article=3096&context=smallsat
      | oppure:
      | -> Sistemare errore in modo che non sia lineare
      | -> Controllare angoli e conversioni
  note: Blocchi per verifica. Quando la flag è positiva errore è nell'inorno di un grado
  DCM_B/N : Inport
  R_N : Inport  Port=2
  Add nose of 1 deg : simulink/Sources/Band-Limited White Noise  Cov=[0.00001 0.00001 0]  Ts=ts_sensor  seed=[23341]
  Asin2 : Trigonometry  Operator=asin
  Asin3 : Trigonometry  Operator=asin
  Constant : Constant  Value=horizon_cone_limit
  Constant1 : Constant  Value=[1 1 1]
  Display{,1..2,5} (4 alike) : Display
  Dot Product2 : DotProduct  OutDataTypeStr=Inherit: Inherit via internal rule
  Dot Product3 : DotProduct  OutDataTypeStr=Inherit: Inherit via internal rule
  Gain : Gain  Gain=-1
  Gain1 : Gain  Gain=-1
  Normalize Vector1 : Subsystem
  Normalize Vector2 : Subsystem
  Perturbed Pitch : Display
  Perturbed Roll : Display
  Radians to Degrees2 : simulink_extras/Transformations/Radians to Degrees
  Radians to Degrees3 : simulink_extras/Transformations/Radians to Degrees
  Rotation in body frame : Product  Multiplication=Matrix(*)
  Rotation in body frame1 : Product  Multiplication=Matrix(*)
  Scope : Scope
  Sum : Sum  Inputs=|++
  Switch : Switch  Criteria=u2 > Threshold  SaturateOnIntegerOverflow=off  InputSameDT=off
  True Roll and Pitch betwen nadir and -z_body : Subsystem
  Unit Delay : UnitDelay  InitialCondition=[0 1 0]'  SampleTime=-1  HasFrameUpgradeWarning=on
  Zero-Order Hold : ZeroOrderHold  SampleTime=ts_sensor
  x_b in body frame2 : Constant  Value=[1,0,0]'
  y_b in body frame3 : Constant  Value=[0,1,0]'
  Perturbed data Horizon : Outport
  R_N Horizon : Outport  Port=2
  Falg IsEarthVisible : Outport  Port=3
  wires:
  y_b in body frame3/1 -> Dot Product3/1
  Zero-Order Hold/1 -> Rotation in body frame1/2
  True Roll and Pitch betwen nadir and -z_body/3(Flag SensorSeeEarth) -> Falg IsEarthVisible/1, Display2/1, Switch/2
  Normalize Vector1/1(Versor) -> Rotation in body frame/2
  Rotation in body frame1/1 -> Sum/1
  Asin2/1 -> Gain/1
  DCM_B/N/1 -> Rotation in body frame/1, Rotation in body frame1/1
  Switch/1 -> Unit Delay/1, Display5/1
  True Roll and Pitch betwen nadir and -z_body/1(Pitch) -> Display/1
  Constant/1 -> True Roll and Pitch betwen nadir and -z_body/1(cone_limit_angle)
  Dot Product2/1 -> Asin2/1
  Rotation in body frame/1 -> True Roll and Pitch betwen nadir and -z_body/2(R_b)  "R_b unperturbed body frame"
  Add nose of 1 deg/1 -> Sum/2
  True Roll and Pitch betwen nadir and -z_body/2(Roll) -> Display1/1
  x_b in body frame2/1 -> Dot Product2/1
  Radians to Degrees2/1 -> Perturbed Pitch/1
  Sum/1 -> Scope/1, Switch/1, Normalize Vector2/1(Vector)
  Dot Product3/1 -> Asin3/1
  Asin3/1 -> Radians to Degrees3/1
  Gain/1 -> Radians to Degrees2/1
  Radians to Degrees3/1 -> Perturbed Roll/1
  Constant1/1 -> Switch/3
  R_N/1 -> Gain1/1  "R_N Sat Earth vector"
  Normalize Vector2/1(Versor) -> Dot Product2/2, Dot Product3/2
  Gain1/1 -> Zero-Order Hold/1, Normalize Vector1/1(Vector), R_N Horizon/1
  Unit Delay/1 -> Perturbed data Horizon/1

== system SAD_projectSamu/Attitude determination and sensoring/MAG-3  Magnetometer1 ==
  note: CODE TO ADD TO MAKE SENSOR WORK
      | % Time definition
      | t0 = 0;
      | tf = T; %Period of orbit
      | t_step = 0.01; %fixed step of simulation
      | ts_sensor = t_step; % Sample of sensor (can change but must to be a multiple of t_step)
      |
      | % MAG-3 sensor data and error
      | FS = 500e-9; %Full scale value
      | inc_lin = 0.15/100; % Accuracy error
      | inc_acc = 0.75/100; % Linear error
      | inc_tot = sqrt(inc_lin^2 + inc_acc^2); %Total error
  DCM_B/N : Inport
  B_N : Inport  Port=2
  Error gain of sensor MAG-3 : Gain  Gain=inc_tot*FS
  Rotation in body frame : Product  Multiplication=Matrix(*)
  Saturation to FS : Saturate  UpperLimit=FS  LowerLimit=-FS
  Sum : Sum  Inputs=|++
  Unit Delay : UnitDelay  InitialCondition=[0,0,1]'  SampleTime=-1  HasFrameUpgradeWarning=on
  Vector Concatenate : Concatenate  NumInputs=3
  White Noise : RandomNumber  DisableCoverage=on  Seed=1  SampleTime=ts_sensor
  White Noise1 : RandomNumber  DisableCoverage=on  Seed=2  SampleTime=ts_sensor
  White Noise2 : RandomNumber  DisableCoverage=on  Seed=3  SampleTime=ts_sensor
  Zero-Order Hold : ZeroOrderHold  SampleTime=ts_sensor
  B_b perturbed sensor : Outport
  B_n : Outport  Port=2
  wires:
  Vector Concatenate/1 -> Error gain of sensor MAG-3/1
  White Noise/1 -> Vector Concatenate/1
  Error gain of sensor MAG-3/1 -> Sum/2
  White Noise2/1 -> Vector Concatenate/3
  White Noise1/1 -> Vector Concatenate/2
  DCM_B/N/1 -> Rotation in body frame/1
  B_N/1 -> B_n/1, Zero-Order Hold/1
  Saturation to FS/1 -> Unit Delay/1
  Rotation in body frame/1 -> Sum/1
  Sum/1 -> Saturation to FS/1
  Zero-Order Hold/1 -> Rotation in body frame/2
  Unit Delay/1 -> B_b perturbed sensor/1

== system SAD_projectSamu/Attitude determination and sensoring/Relative attitude error quaternion2 ==
  q1 (usually Target) : Inport
  q2 (Estimated) : Inport  Port=2
  Demux : Demux
  Gain1 : Gain  Gain=[0,0,0,-1; 0,0,1,0; 0,-1,0 0; 1,0,0,0]
  Gain2 : Gain  Gain=[0, 0, -1 ,0; 0, 0 ,0 ,-1; 1, 0, 0, 0; 0 1, 0, 0]
  Gain3 : Gain  Gain=[0 1 0 0; -1 0 0 0; 0 0 0 -1; 0 0 1 0]
  Gain4 : Gain  Gain=eye(4)
  Matrix Multiply : Product  Multiplication=Matrix(*)
  Sum1 : Sum  Inputs=++++
  qe : Outport
  wires:
  Gain1/1 -> Sum1/1
  Demux/2 -> Gain2/1
  Gain3/1 -> Sum1/3
  Demux/1 -> Gain1/1
  Sum1/1 -> Matrix Multiply/1
  Demux/3 -> Gain3/1
  Gain4/1 -> Sum1/4
  Gain2/1 -> Sum1/2
  Demux/4 -> Gain4/1
  q2 (Estimated)/1 -> Matrix Multiply/2
  Matrix Multiply/1 -> qe/1
  q1 (usually Target)/1 -> Demux/1

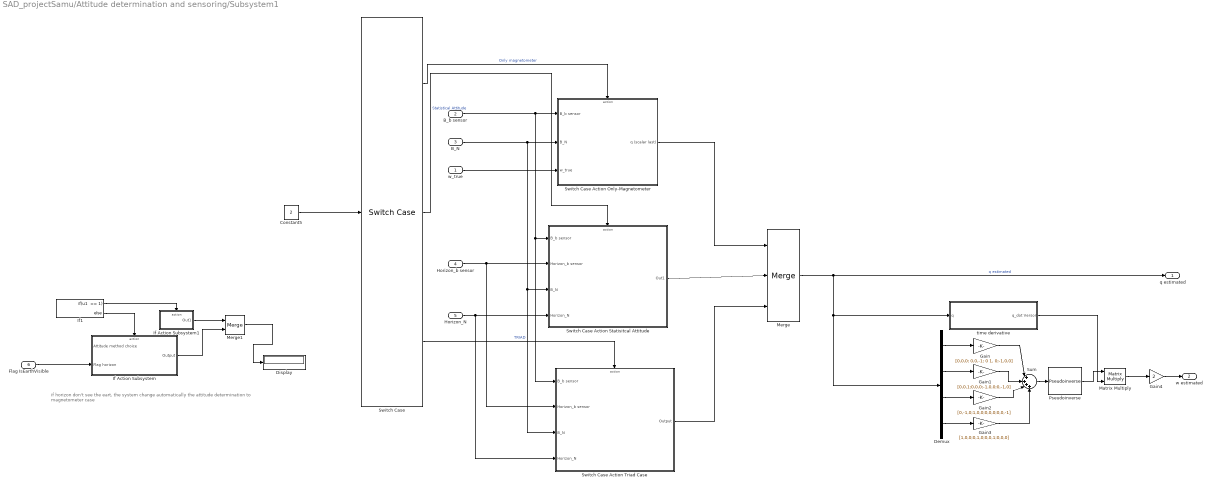
== system SAD_projectSamu/Attitude determination and sensoring/Subsystem1 ==
  note: if horizon don't see the eart, the system change automatically the attitude determination to magnetometer case
  w_true : Inport
  B_b sensor : Inport  Port=2
  B_N : Inport  Port=3
  Horizon_b sensor : Inport  Port=4
  Horizon_N : Inport  Port=5
  Flag IsEarthVisible : Inport  Port=6
  Constant5 : Constant  Value=2
  Demux : Demux
  Display : Display
  Gain : Gain  Gain=[0,0,0; 0,0,-1; 0 1, 0;-1,0,0]
  Gain1 : Gain  Gain=[0,0,1;0,0,0;-1,0,0;0,-1,0]
  Gain2 : Gain  Gain=[0,-1,0;1,0,0;0,0,0;0,0,-1]
  Gain3 : Gain  Gain=[1,0,0;0,1,0;0,0,1;0,0,0]
  Gain4 : Gain  Gain=2
  If Action Subsystem : Subsystem  TreatAsAtomicUnit=on
  If Action Subsystem1 : Subsystem  TreatAsAtomicUnit=on
  If1 : If  IfExpression="u1  == 1"
  Matrix Multiply : Product  Multiplication=Matrix(*)
  Merge : Merge  Inputs=3
  Merge1 : Merge
  Pseudoinverse : dspinverses/Pseudoinverse  wanterr=off  SimulateUsing=Interpreted execution
  Sum : Sum  Inputs=|++++
  Switch Case : SwitchCase  CaseConditions={1,2}
  Switch Case Action Only-Magnetometer : Subsystem  TreatAsAtomicUnit=on
  Switch Case Action Statisitcal Attitude : Subsystem  TreatAsAtomicUnit=on
  Switch Case Action Triad Case : Subsystem  TreatAsAtomicUnit=on
  time derivative : Subsystem
  q estimated : Outport
  w estimated : Outport  Port=2
  wires:
  Switch Case/3 -> Switch Case Action Triad Case/Action  "TRIAD"
  Switch Case Action Statisitcal Attitude/1(Out1) -> Merge/2
  Switch Case Action Triad Case/1(Output) -> Merge/3
  Switch Case/2 -> Switch Case Action Statisitcal Attitude/Action  "Statistical Attitude"
  Switch Case Action Only-Magnetometer/1(q (scalar last)) -> Merge/1
  Switch Case/1 -> Switch Case Action Only-Magnetometer/Action  "Only magnetometer"
  Merge/1 -> q estimated/1, time derivative/1(q), Demux/1  "q estimated"
  w_true/1 -> Switch Case Action Only-Magnetometer/3(w_true)
  Horizon_b sensor/1 -> Switch Case Action Statisitcal Attitude/2(Horizon_b sensor), Switch Case Action Triad Case/2(Horizon_b sensor)
  Horizon_N/1 -> Switch Case Action Triad Case/4(Horizon_N), Switch Case Action Statisitcal Attitude/4(Horizon_N)
  B_N/1 -> Switch Case Action Only-Magnetometer/2(B_N), Switch Case Action Triad Case/3(B_N), Switch Case Action Statisitcal Attitude/3(B_N)
  B_b sensor/1 -> Switch Case Action Only-Magnetometer/1(B_b sensor), Switch Case Action Triad Case/1(B_b sensor), Switch Case Action Statisitcal Attitude/1(B_b sensor)
  If1/2 -> If Action Subsystem/Action
  Flag IsEarthVisible/1 -> If Action Subsystem/2(Flag horizon)
  If Action Subsystem/1(Output) -> Merge1/2
  Merge1/1 -> Display/1
  If1/1 -> If Action Subsystem1/Action
  If Action Subsystem1/1(Out1) -> Merge1/1
  Demux/1 -> Gain/1
  Demux/2 -> Gain1/1
  Demux/3 -> Gain2/1
  Demux/4 -> Gain3/1
  Gain/1 -> Sum/1
  Gain1/1 -> Sum/2
  Gain2/1 -> Sum/3
  Gain3/1 -> Sum/4
  Matrix Multiply/1 -> Gain4/1
  Sum/1 -> Pseudoinverse/1
  Gain4/1 -> w estimated/1
  Pseudoinverse/1 -> Matrix Multiply/1
  time derivative/1(q_dot Versor) -> Matrix Multiply/2
  Constant5/1 -> Switch Case/1

== system SAD_projectSamu/Calculation of disturbance torque/M of gravity gradient1 ==
  Inertia Vector : Inport
  A_B/L : Inport  Port=2
  r_N : Inport  Port=3
  Constant : Constant  Value=3
  Constant11 : Constant  Value=[1,0,0]
  Demux1 : Demux  Outputs=3
  Divide : Product  Inputs=*/
  Gain : Gain  Gain=3*mu_E
  Gain1 : Gain  Gain=[0;-1;1]
  Gain2 : Gain  Gain=[1;0;-1]
  Gain3 : Gain  Gain=[-1;1;0]
  Matrix Multiply2 : Product  Multiplication=Matrix(*)
  Norm of vector : Subsystem  AncestorBlock=LibrarySAD5/Normalize Vector1
  Power : Math  Operator=pow
  Product2 : Product  Inputs=3
  Product3 : Product  Inputs=3
  Product4 : Product  Inputs=3
  Scope : Scope
  Sum of Elements : Sum  Inputs=+
  Sum of Elements1 : Sum  Inputs=+
  Sum of Elements2 : Sum  Inputs=+
  Vector Concatenate4 : Concatenate  NumInputs=3
  GravityGradient_M : Outport
  wires:
  Demux1/3 -> Product2/3, Product3/3
  Product2/1 -> Vector Concatenate4/1
  Matrix Multiply2/1 -> Demux1/1
  Product4/1 -> Vector Concatenate4/3
  Product3/1 -> Vector Concatenate4/2
  Demux1/1 -> Product4/2, Product3/2
  Constant11/1 -> Matrix Multiply2/2
  Demux1/2 -> Product4/3, Product2/2
  A_B/L/1 -> Matrix Multiply2/1
  Vector Concatenate4/1 -> Gain/1
  Gain1/1 -> Sum of Elements/1
  Gain2/1 -> Sum of Elements1/1
  Gain3/1 -> Sum of Elements2/1
  Sum of Elements/1 -> Product2/1
  Sum of Elements1/1 -> Product3/1
  Sum of Elements2/1 -> Product4/1
  Inertia Vector/1 -> Gain1/1, Gain2/1, Gain3/1
  Gain/1 -> Divide/1
  Power/1 -> Scope/1, Divide/2
  Constant/1 -> Power/2
  r_N/1 -> Norm of vector/1(Vector)
  Divide/1 -> GravityGradient_M/1
  Norm of vector/1(Norm) -> Power/1

== system SAD_projectSamu/Calculation of disturbance torque/Magnetic Torque ==
  j_b : Inport
  B_b : Inport  Port=2
  Cross Product : matrix_library/Cross Product
  M_b : Outport
  wires:
  Cross Product/1 -> M_b/1
  j_b/1 -> Cross Product/1
  B_b/1 -> Cross Product/2

== system SAD_projectSamu/Calculation of disturbance torque/Solar pressure on 6 faces ==
  DCM_BN : Inport
  "r_N " : Inport  Port=2
  S_N : Inport  Port=3
  Acos : Trigonometry  Operator=acos
  Dot Product : DotProduct  OutDataTypeStr=Inherit: Inherit via internal rule
  MatrixMultiply : Product  Multiplication=Matrix(*)
  MatrixMultiply1 : Product  Multiplication=Matrix(*)
  Norm of vector : Subsystem  AncestorBlock=LibrarySAD5/Normalize Vector1
  Normalize Vector : vrlib/Utilities/Normalize Vector  maxzero=0
  Normalize Vector1 : vrlib/Utilities/Normalize Vector  maxzero=0
  Solar pressure on 6 faces1 : Subsystem
  Sum1 : Sum  Inputs=|+-
  Mtot_SP : Outport
  Ftot_SP : Outport  Port=2
  wires:
  DCM_BN/1 -> MatrixMultiply1/1, MatrixMultiply/1
  S_N/1 -> Norm of vector/1(Vector), Sum1/1, MatrixMultiply/2, Normalize Vector1/1
  "r_N "/1 -> Sum1/2, MatrixMultiply1/2
  MatrixMultiply1/1 -> Solar pressure on 6 faces1/2(r_B)
  Norm of vector/1(Norm) -> Solar pressure on 6 faces1/5(s_N norm)
  MatrixMultiply/1 -> Solar pressure on 6 faces1/1(s_B)
  Sum1/1 -> Solar pressure on 6 faces1/4(S_N - r_N), Normalize Vector/1
  Normalize Vector/1 -> Dot Product/1
  Normalize Vector1/1 -> Dot Product/2
  Solar pressure on 6 faces1/1(Ftot_SP) -> Ftot_SP/1
  Dot Product/1 -> Acos/1
  Acos/1 -> Solar pressure on 6 faces1/3(S/E_S/sc_angle)
  Solar pressure on 6 faces1/2(Mtot_SP) -> Mtot_SP/1

== system SAD_projectSamu/Create matrix to statistical method/Normalize Vector1 ==
  Vector : Inport
  Divide : Product  Inputs=*/
  Normalize Vector : Subsystem  AncestorBlock=LibrarySAD5/Normalize Vector1
  Versor : Outport
  wires:
  Vector/1 -> Normalize Vector/1(Vector), Divide/1
  Divide/1 -> Versor/1
  Normalize Vector/1(Norm) -> Divide/2

== system SAD_projectSamu/Create matrix to statistical method/Normalize Vector2 ==
  Vector : Inport
  Divide : Product  Inputs=*/
  Normalize Vector : Subsystem  AncestorBlock=LibrarySAD5/Normalize Vector1
  Versor : Outport
  wires:
  Vector/1 -> Normalize Vector/1(Vector), Divide/1
  Divide/1 -> Versor/1
  Normalize Vector/1(Norm) -> Divide/2

== system SAD_projectSamu/Create matrix to statistical method/Normalize Vector3 ==
  Vector : Inport
  Divide : Product  Inputs=*/
  Normalize Vector : Subsystem  AncestorBlock=LibrarySAD5/Normalize Vector1
  Versor : Outport
  wires:
  Vector/1 -> Normalize Vector/1(Vector), Divide/1
  Divide/1 -> Versor/1
  Normalize Vector/1(Norm) -> Divide/2

== system SAD_projectSamu/Create matrix to statistical method/Normalize Vector4 ==
  Vector : Inport
  Divide : Product  Inputs=*/
  Normalize Vector : Subsystem  AncestorBlock=LibrarySAD5/Normalize Vector1
  Versor : Outport
  wires:
  Vector/1 -> Normalize Vector/1(Vector), Divide/1
  Divide/1 -> Versor/1
  Normalize Vector/1(Norm) -> Divide/2

== system SAD_projectSamu/DCM to quaternion/Normalize Vector1 ==
  Vector : Inport
  Divide : Product  Inputs=*/
  Norm vector : Subsystem  AncestorBlock=LibrarySAD5/Normalize Vector1
  Versor : Outport
  wires:
  Vector/1 -> Norm vector/1(Vector), Divide/1
  Divide/1 -> Versor/1
  Norm vector/1(Norm) -> Divide/2

== system SAD_projectSamu/Determine Control algorithm/Relative attitude error quaternion3 ==
  q1 (usually Target) : Inport
  q2 (Estimated) : Inport  Port=2
  Demux : Demux
  Gain1 : Gain  Gain=[0,0,0,-1; 0,0,1,0; 0,-1,0 0; 1,0,0,0]
  Gain2 : Gain  Gain=[0, 0, -1 ,0; 0, 0 ,0 ,-1; 1, 0, 0, 0; 0 1, 0, 0]
  Gain3 : Gain  Gain=[0 1 0 0; -1 0 0 0; 0 0 0 -1; 0 0 1 0]
  Gain4 : Gain  Gain=eye(4)
  Matrix Multiply : Product  Multiplication=Matrix(*)
  Sum1 : Sum  Inputs=++++
  Zero-Order Hold1 : ZeroOrderHold  SampleTime=5*ts_sensor
  qe : Outport
  wires:
  Gain1/1 -> Sum1/1
  Demux/2 -> Gain2/1
  Gain3/1 -> Sum1/3
  Demux/1 -> Gain1/1
  Sum1/1 -> Matrix Multiply/1
  Demux/3 -> Gain3/1
  Gain4/1 -> Sum1/4
  Gain2/1 -> Sum1/2
  Demux/4 -> Gain4/1
  q2 (Estimated)/1 -> Matrix Multiply/2
  Matrix Multiply/1 -> qe/1
  q1 (usually Target)/1 -> Zero-Order Hold1/1
  Zero-Order Hold1/1 -> Demux/1

== system SAD_projectSamu/Determine Control algorithm/Switch Case Action 3 axis stabilization Algorithm ==
  note: teoria presa da bernelli pt 3 pag 52
  BusElementIn : Inport  PortName=Model info  Element=A_L/N
  BusElementIn2 : Inport  Port=2  PortName=InBus  Element=q estimated
  BusElementIn3 : Inport  Port=2  PortName=InBus  Element=w estimated
  Action Port : ActionPort  ActionPortLabel=case [ 3 ]:
  Constant : Constant  Value=[0,0,0]'
  Constant1 : Constant  Value=-K2_point
  Constant2 : Constant  Value=K1_point
  DCM to quaternion1 : Subsystem
  Demux1 : Demux
  IsNaN : RelationalOperator  Operator=isNaN  OutDataTypeStr=boolean  RndMeth=Simplest  InputSameDT=off
  Matrix Multiply1 : Product  Multiplication=Matrix(*)
  Matrix Multiply2 : Product  Multiplication=Matrix(*)
  Norm vector : Subsystem  AncestorBlock=LibrarySAD5/Normalize Vector1
  Product2 : Product
  Relative attitude error quaternion3 : Subsystem
  Sum1 : Sum  Inputs=|+-
  Switch : Switch  Criteria=u2 > Threshold  SaturateOnIntegerOverflow=off  InputSameDT=off
  Vector Concatenate1 : Concatenate  NumInputs=3
  Mc : Outport
  q target : Outport  Port=2
  wires:
  Demux1/1 -> Vector Concatenate1/1
  BusElementIn2/1 -> Relative attitude error quaternion3/2(q2 (Estimated))
  BusElementIn/1 -> DCM to quaternion1/1(DCM)
  Relative attitude error quaternion3/1(qe) -> Demux1/1
  Matrix Multiply1/1 -> Product2/1
  DCM to quaternion1/1(q (scalar last)1) -> q target/1, Relative attitude error quaternion3/1(q1 (usually Target))
  Demux1/2 -> Vector Concatenate1/2
  Demux1/3 -> Vector Concatenate1/3
  Demux1/4 -> Product2/2
  Constant/1 -> Switch/1
  Constant2/1 -> Matrix Multiply2/1
  Constant1/1 -> Matrix Multiply1/1
  Vector Concatenate1/1 -> Matrix Multiply1/2
  BusElementIn3/1 -> Matrix Multiply2/2
  Product2/1 -> Sum1/1
  Matrix Multiply2/1 -> Sum1/2
  Sum1/1 -> Switch/3, IsNaN/1
  IsNaN/1 -> Norm vector/1(Vector)
  Switch/1 -> Mc/1
  Norm vector/1(Norm) -> Switch/2
